simulink model "simModel2020"  (R2023b)
settings: Solver=ode4  StartTime=0  StopTime=360  FixedStep=0.01  RelTol=1e-3
values from neighbouring files (symbols this model uses):
  B747 =     [B747.mat]
undefined symbols (not defined in the file or in its folder): airport, APP, control, Curise, Earth, env, ft, m, navData, navParam, Newton, plotTrack, Raphson, s, TakeOff, WGS84
libraries: aerolibconvert2 x18, simulink x15, sharedtransform x4, aerolibfltsims x3, aerolibatmos2 x2, shared6dof x2, aerolibasang x2, dspsrcs4 x2, aerolibwind2 x2, aerolibanimutils x1, aerolibpropulsion2 x1, aerolibtransform2 x1
(part 2 of 6)

== system simModel2020/PlantModel/Actuator Model/Linear Second-Order Actuator4 ==
  Ac_dem : Inport
  2*zeta * wn : Gain  Gain=2.0 * z_fin* wn_fin  SaturateOnIntegerOverflow=on  OutDataTypeStr=Inherit: Same as input  ParamDataTypeStr=Inherit: Same as input
  "Integrator, Second-Order" : SecondOrderIntegrator  ICX=fin_act_0  UpperLimitX=1  LowerLimitX=0  ICDXDT=fin_act_vel
  Sum2 : Sum  Inputs=|+-  InputSameDT=on  SaturateOnIntegerOverflow=on  OutDataTypeStr=Inherit: Same as first input
  Sum3 : Sum  Inputs=|+-  InputSameDT=on  SaturateOnIntegerOverflow=on  OutDataTypeStr=Inherit: Same as first input
  wn^2 : Gain  Gain=wn_fin* wn_fin  SaturateOnIntegerOverflow=on  OutDataTypeStr=Inherit: Same as input  ParamDataTypeStr=Inherit: Same as input
  Ac_ac : Outport  InitialOutput=0
  wires:
  "Integrator, Second-Order"/1 -> Ac_ac/1, Sum3/2
  wn^2/1 -> Sum2/1
  Sum2/1 -> "Integrator, Second-Order"/1
  2*zeta * wn/1 -> Sum2/2
  Ac_dem/1 -> Sum3/1
  Sum3/1 -> wn^2/1
  "Integrator, Second-Order"/2 -> 2*zeta * wn/1

== system simModel2020/PlantModel/B747 Dynamics动力学参数计算/6DOF Equations of Motion运动学方程 ==
  note: 此处vb为地速ve进行坐标转换得到
  FM_b : Inport
  oil Q : Inport  Port=2
  IsGround : Inport  Port=3
  Deviation On : Inport  Port=4
  6DOF (Euler Angles) : shared6dof/6DOF (Euler Angles)  units=Metric (MKS)  mtype=Fixed  rep=Euler Angles  xme_0=[0 0 0]  Vm_0=[0 0 0]  eul_0=[0 0 0]  pm_0=[0 0 0]  mass_0=1.0  mass_e=0.5  mass_f=2.0  inertia=eye(3)  inertia_e=eye(3)  inertia_f=2*eye(3)  k_quat=1.0  vre_flag=on  abi_flag=off  aMode=0  xme_statename=''  Vm_statename=''  eul_statename=''  quat_statename=''  pm_statename=''  mass_statename=''
  6DOF (Euler Angles)1 : shared6dof/6DOF (Euler Angles)  units=Metric (MKS)  mtype=Simple Variable  rep=Euler Angles  xme_0=B747.ic.Pos_0.*[1; 1; -1]  Vm_0=B747.ic.Vb_0  eul_0=B747.ic.Euler_0  pm_0=B747.ic.PQR_0  mass_0=B747.geometry.mass  mass_e=B747.geometry.massEmpty  mass_f=B747.geometry.massFull  inertia=eye(3)  inertia_e=diag([B747.inertia.Ixx B747.inertia.Iyy B747.inertia.Izz])  inertia_f=diag([B747.inertia.Ixx B747.inertia.Iyy B747.inertia.Izz])  k_quat=1.0  vre_flag=off  abi_flag=off  aMode=aMode  xme_statename=''  Vm_statename=''  eul_statename=''  quat_statename=''  pm_statename=''  mass_statename=''
  Bus Creator : BusCreator  Inputs=8
  Compute psi_dot : Subsystem
  Constant1 : Constant  Value=0
  Demux2 : Demux  Outputs=2
  Multiport Switch : MultiPortSwitch  DataPortOrder=Specify indices  Inputs=[0 1]  DataPortIndices={1,0}  SaturateOnIntegerOverflow=off  InputSameDT=off
  Terminator : Terminator
  Terminator1 : Terminator
  Terminator2 : Terminator
  To Workspace : ToWorkspace  VariableName=Fuel  SampleTime=-1
  "[0, pi] Wrap Around" : Subsystem
  B747 State : Outport
  wires:
  6DOF (Euler Angles)1/8 -> Bus Creator/6  "Ab"
  "[0, pi] Wrap Around"/1(Wrapped) -> Bus Creator/3  "Euler"
  6DOF (Euler Angles)1/5 -> Bus Creator/4  "Vb"
  6DOF (Euler Angles)1/2 -> Bus Creator/2  "Xe"
  6DOF (Euler Angles)1/1 -> Bus Creator/1  "Ve"
  Bus Creator/1 -> B747 State/1
  6DOF (Euler Angles)1/4 -> Terminator1/1
  6DOF (Euler Angles)1/3 -> Compute psi_dot/1(Euler), "[0, pi] Wrap Around"/1(Euler)
  6DOF (Euler Angles)1/6 -> Compute psi_dot/2(G), Bus Creator/5  "pqr"
  FM_b/1 -> Demux2/1
  Demux2/1 -> 6DOF (Euler Angles)1/1
  Compute psi_dot/1(psi_dot) -> Bus Creator/7  "psi_dot"
  Demux2/2 -> 6DOF (Euler Angles)1/2
  Multiport Switch/1 -> 6DOF (Euler Angles)1/3
  Constant1/1 -> Multiport Switch/3
  Deviation On/1 -> Multiport Switch/1
  oil Q/1 -> Multiport Switch/2
  6DOF (Euler Angles)1/9 -> To Workspace/1, Terminator/1
  6DOF (Euler Angles)1/7 -> Terminator2/1
  IsGround/1 -> Bus Creator/8  "IsGround"

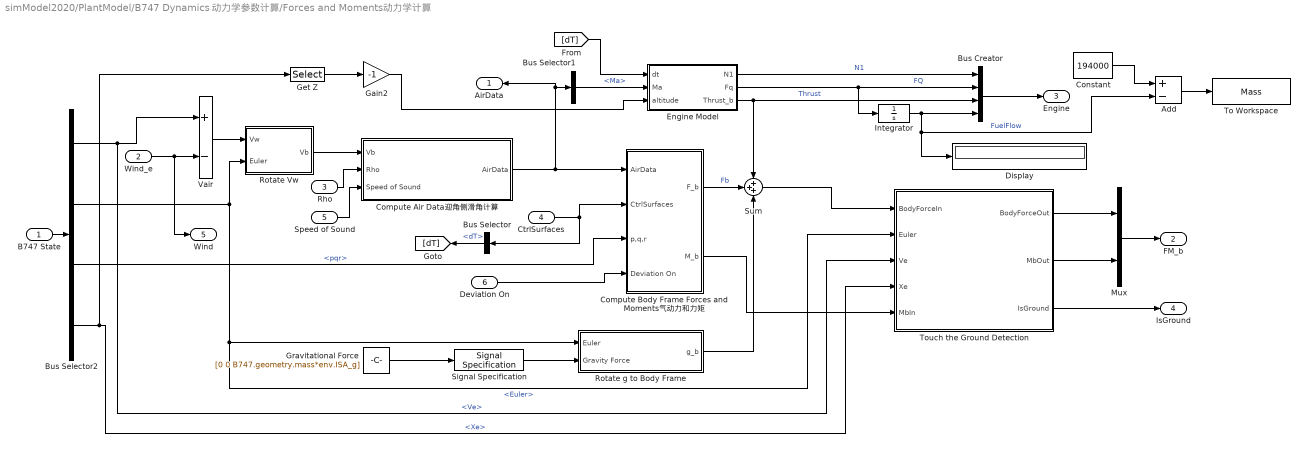
== system simModel2020/PlantModel/B747 Dynamics动力学参数计算/Forces and Moments动力学计算 ==
  B747 State : Inport
  Wind_e : Inport  Port=2
  Rho : Inport  Port=3
  CtrlSurfaces : Inport  Port=4
  Speed of Sound : Inport  Port=5
  Deviation On : Inport  Port=6
  Add : Sum  Inputs=+-
  Bus Creator : BusCreator  Inputs=4
  Bus Selector : BusSelector  OutputSignals=dT
  Bus Selector1 : BusSelector  OutputSignals=Ma
  Bus Selector2 : BusSelector  OutputSignals=Ve,Euler,pqr,Xe
  Compute Air Data迎角侧滑角计算 : Subsystem  TreatAsAtomicUnit=on  VariantControl=use_aerospace_blocks == 1
  Compute Body Frame Forces and Moments气动力和力矩 : Subsystem
  Constant : Constant  Value=194000
  Display : Display
  Engine Model : Subsystem
  Gain2 : Gain  Gain=-1
      settings: AttributesFormatString=Z to Alt
  Get Z : Selector  InputPortWidth=3  IndexOptions=Index vector (dialog)  Indices=[3]  OutputSizes=[(-2)]
  Gravitational Force : Constant  Value=[0 0 B747.geometry.mass*env.ISA_g]  VectorParams1D=off
      settings: AttributesFormatString=%<Value>
  Integrator : Integrator
  Mux : Mux  Inputs=2
  Rotate Vw : Subsystem
  Rotate g to Body Frame : Subsystem
  Signal Specification : SignalSpecification
  Sum : Sum  Inputs=+++  SaturateOnIntegerOverflow=on
  To Workspace : ToWorkspace  VariableName=Mass  SampleTime=-1
  Touch the Ground Detection : Subsystem
  Vair : Sum  Inputs=+-  InputSameDT=on  SaturateOnIntegerOverflow=on  OutDataTypeStr=Inherit: Same as first input
  AirData : Outport
  FM_b : Outport  Port=2
  Engine : Outport  Port=3
  IsGround : Outport  Port=4
  Wind : Outport  Port=5
  wires:
  Bus Selector2/1 -> Touch the Ground Detection/3(Ve), Vair/1  "<Ve>"
  B747 State/1 -> Bus Selector2/1
  Mux/1 -> FM_b/1
  Bus Selector/1 -> [dT]  "<dT>"
  Compute Body Frame Forces and Moments气动力和力矩/1(F_b) -> Sum/2  "Fb"
  Rotate g to Body Frame/1(g_b) -> Sum/3
  Wind_e/1 -> Wind/1, Vair/2
  CtrlSurfaces/1 -> Compute Body Frame Forces and Moments气动力和力矩/2(CtrlSurfaces), Bus Selector/1
  Bus Selector2/3 -> Compute Body Frame Forces and Moments气动力和力矩/3(p,q,r)  "<pqr>"
  Gravitational Force/1 -> Signal Specification/1
  Rotate Vw/1(Vb) -> Compute Air Data迎角侧滑角计算/1(Vb)
  Rho/1 -> Compute Air Data迎角侧滑角计算/2(Rho)
  Bus Selector2/2 -> Rotate Vw/2(Euler), Touch the Ground Detection/2(Euler), Rotate g to Body Frame/1(Euler)  "<Euler>"
  Vair/1 -> Rotate Vw/1(Vw)
  Signal Specification/1 -> Rotate g to Body Frame/2(Gravity Force)
  Touch the Ground Detection/1(BodyForceOut) -> Mux/1
  Sum/1 -> Touch the Ground Detection/1(BodyForceIn)
  Compute Body Frame Forces and Moments气动力和力矩/2(M_b) -> Touch the Ground Detection/5(MbIn)
  Touch the Ground Detection/2(MbOut) -> Mux/2
  Speed of Sound/1 -> Compute Air Data迎角侧滑角计算/3(Speed of Sound)
  Engine Model/1(N1) -> Bus Creator/1  "N1"
  [dT] -> Engine Model/1(dt)
  Engine Model/2(Fq) -> Integrator/1, Bus Creator/2  "FQ"
  Get Z/1 -> Gain2/1
  Bus Selector2/4 -> Get Z/1, Touch the Ground Detection/4(Xe)  "<Xe>"
  Compute Air Data迎角侧滑角计算/1(AirData) -> AirData/1, Bus Selector1/1, Compute Body Frame Forces and Moments气动力和力矩/1(AirData)
  Engine Model/3(Thrust_b) -> Sum/1, Bus Creator/3  "Thrust"
  Bus Selector1/1 -> Engine Model/2(Ma)  "<Ma>"
  Gain2/1 -> Engine Model/3(altitude)
  Deviation On/1 -> Compute Body Frame Forces and Moments气动力和力矩/4(Deviation On)
  Bus Creator/1 -> Engine/1
  Integrator/1 -> Bus Creator/4, Display/1, Add/2  "FuelFlow"
  Touch the Ground Detection/3(IsGround) -> IsGround/1
  Constant/1 -> Add/1
  Add/1 -> To Workspace/1

== system simModel2020/PlantModel/FlightSwitchModel/If Action Subsystem ==
  In1 : Inport
  Action Port : ActionPort  ActionPortLabel=case [ 2 ]:
  Out1 : Outport
  wires:
  In1/1 -> Out1/1

== system simModel2020/PlantModel/FlightSwitchModel/If Action Subsystem1 ==
  CtrlCmds : Inport
  Action Port : ActionPort  ActionPortLabel=case [ 0 ]:
  Out1 : Outport
  wires:
  CtrlCmds/1 -> Out1/1

== system simModel2020/PlantModel/FlightSwitchModel/If Action Subsystem2 ==
  CtrlCmds : Inport
  Action Port : ActionPort  ActionPortLabel=case [ 1 ]:
  Out1 : Outport
  wires:
  CtrlCmds/1 -> Out1/1

== system simModel2020/PlantModel/FlightSwitchModel/Manually piloted aircraft ==
  Gain : Gain  Gain=pi/180
  Gain1 : Gain  Gain=1/100
  Gain2 : Gain  Gain=pi/180
  Gain3 : Gain  Gain=pi/180
  Mux : Mux  Inputs=5
  dA_hand : Constant  Value=16.8
  dE_hand : Constant  Value=-17.3643
  dF_hand : Constant  Value=0
  dR_hand : Constant  Value=-1.3333
  dT_hand : Constant  Value=65.1111
  Out1 : Outport
  wires:
  Mux/1 -> Out1/1
  dR_hand/1 -> Gain3/1
  dA_hand/1 -> Gain2/1
  dE_hand/1 -> Gain/1
  dT_hand/1 -> Gain1/1
  dF_hand/1 -> Mux/5
  Gain/1 -> Mux/1
  Gain1/1 -> Mux/2
  Gain2/1 -> Mux/3
  Gain3/1 -> Mux/4

== system simModel2020/PlantModel/Sensor Model/Assemble GPS and State Data ==
  AirSensorData : Inport
  B747 State : Inport  Port=2
  CtrlSurfaces : Inport  Port=3
  Engine : Inport  Port=4
  Wind : Inport  Port=5
  Bus Creator : BusCreator  Inputs=20
  Bus Selector : BusSelector  OutputSignals=static,q,OAT,airpseed,alpha,beta,Ma,ias
  Bus Selector1 : BusSelector  OutputSignals=dE,dT,dA,dR,dF
  Bus Selector2 : BusSelector  OutputSignals=Euler,pqr,Xe,Ve,Ab,IsGround,Vb
  Bus Selector3 : BusSelector  OutputSignals=Xe
  Bus Selector5 : BusSelector  OutputSignals=N1,FQ
  LLA Position : Subsystem
  Mux : Mux  Inputs=5
  B747 StateBus : Outport
  wires:
  Mux/1 -> Bus Creator/17  "ctrlSurfacePos"
  CtrlSurfaces/1 -> Bus Selector1/1  "ctrlSurfacePos"
  Bus Selector/4 -> Bus Creator/11  "<airpseed>"
  Bus Selector/3 -> Bus Creator/10  "<OAT>"
  Bus Selector/2 -> Bus Creator/9  "<q>"
  Bus Selector/1 -> Bus Creator/8  "<static>"
  Bus Selector2/5 -> Bus Creator/5  "<Ab>"
  Bus Selector2/4 -> Bus Creator/4  "<Ve>"
  Bus Selector2/2 -> Bus Creator/2  "<pqr>"
  Bus Selector2/1 -> Bus Creator/1  "<Euler>"
  Bus Creator/1 -> B747 StateBus/1
  B747 State/1 -> Bus Selector2/1, Bus Selector3/1
  Bus Selector3/1 -> LLA Position/1(XYZ (NEU))  "<Xe>"
  AirSensorData/1 -> Bus Selector/1
  Bus Selector2/3 -> Bus Creator/3  "<Xe>"
  Bus Selector/5 -> Bus Creator/12  "<alpha>"
  Bus Selector/6 -> Bus Creator/13  "<beta>"
  Engine/1 -> Bus Selector5/1  "Engine"
  Bus Selector5/1 -> Bus Creator/18  "<N1>"
  Bus Selector5/2 -> Bus Creator/19  "<FQ>"
  Bus Selector/7 -> Bus Creator/14  "<Ma>"
  Bus Selector/8 -> Bus Creator/15  "<ias>"
  Bus Selector2/6 -> Bus Creator/6  "<IsGround>"
  LLA Position/1(LLA) -> Bus Creator/16  "LLA"
  Bus Selector1/1 -> Mux/1  "<dE>"
  Bus Selector1/2 -> Mux/2  "<dT>"
  Bus Selector1/3 -> Mux/3  "<dA>"
  Bus Selector1/4 -> Mux/4  "<dR>"
  Bus Selector1/5 -> Mux/5  "<dF>"
  Bus Selector2/7 -> Bus Creator/7  "<Vb>"
  Wind/1 -> Bus Creator/20  "Wind"

== system simModel2020/PlantModel/Sensor Model/Noise Model ==
  note: 加速度
  note: 指示空速
  note: 经纬高
  note: 燃油速率
  note: 发动机转速
  note: 操纵面位置
  note: 马赫数
  note: 气流角
  note: 真空速
  note: 外界温度
  note: 动压
  note: 静压
  note: 速度
  note: 位置
  note: 角速率
  note: 欧拉角
  B747 State : Inport
  Bus Creator : BusCreator  Inputs=20
  Bus Selector2 : BusSelector  OutputSignals=Euler,pqr,Xe,Ve,Ab,static,q,OAT,airpseed,alpha,beta,Ma,ctrlSurfacePos,N1,FQ,LLA,ias,IsGround,Vb,Wind
  Gain1 : Gain  Gain=[1 1 -1]
  Gain2 : Gain  Gain=[1 1 -1]
  SensorData : Outport
  wires:
  Bus Creator/1 -> SensorData/1
  Bus Selector2/8 -> Bus Creator/8  "<OAT>"
  Bus Selector2/7 -> Bus Creator/7  "<q>"
  Bus Selector2/6 -> Bus Creator/6  "<static>"
  Bus Selector2/4 -> Gain1/1  "<Ve>"
  Bus Selector2/1 -> Bus Creator/1  "<Euler>"
  B747 State/1 -> Bus Selector2/1
  Bus Selector2/10 -> Bus Creator/10  "<alpha>"
  Bus Selector2/3 -> Gain2/1  "<Xe>"
  Bus Selector2/5 -> Bus Creator/5  "<Ab>"
  Bus Selector2/9 -> Bus Creator/9  "<airpseed>"
  Bus Selector2/2 -> Bus Creator/2  "<pqr>"
  Gain2/1 -> Bus Creator/3  "Xe"
  Gain1/1 -> Bus Creator/4  "Ve"
  Bus Selector2/11 -> Bus Creator/11  "<beta>"
  Bus Selector2/12 -> Bus Creator/12  "<Ma>"
  Bus Selector2/13 -> Bus Creator/13  "<ctrlSurfacePos>"
  Bus Selector2/14 -> Bus Creator/14  "<N1>"
  Bus Selector2/15 -> Bus Creator/15  "<FQ>"
  Bus Selector2/16 -> Bus Creator/16  "<LLA>"
  Bus Selector2/17 -> Bus Creator/17  "<ias>"
  Bus Selector2/18 -> Bus Creator/18  "<IsGround>"
  Bus Selector2/19 -> Bus Creator/19  "<Vb>"
  Bus Selector2/20 -> Bus Creator/20  "<Wind>"

== system simModel2020/PlantModel/Wind Model/ Compute Norm ==
  V : Inport
  Dot Product : DotProduct  OutDataTypeStr=Inherit: Inherit via internal rule
  Math Function1 : Sqrt  AlgorithmType=Newton-Raphson
      settings: AttributesFormatString=%<AlgorithmType>
  Zero Bound : Saturate  UpperLimit=inf  LowerLimit=0.001
      settings: AttributesFormatString="[%<LowerLimit>  %<UpperLimit>]"
  |V| : Outport
  wires:
  Math Function1/1 -> |V|/1
  V/1 -> Dot Product/2, Dot Product/1
  Dot Product/1 -> Zero Bound/1
  Zero Bound/1 -> Math Function1/1

== system simModel2020/PlantModel/Wind Model/Average wind ==
  DCM : Inport
  " " : Gain  Gain=-1  SaturateOnIntegerOverflow=on  OutDataTypeStr=Inherit: Same as input  ParamDataTypeStr=Inherit: Same as input
  Angle Conversion : aerolibconvert2/Angle Conversion  IU=deg  OU=rad
  Mux : Mux  Inputs=3
  Product1 : Product  InputSameDT=on  SaturateOnIntegerOverflow=on  OutDataTypeStr=Inherit: Same as first input
  SinCos : Trigonometry  Operator=sincos
  Transform from Inertial to Body axes : Product  Inputs=**  Multiplication=Matrix(*)  InputSameDT=on  SaturateOnIntegerOverflow=on  OutDataTypeStr=Inherit: Same as first input
  Wdeg1 : Constant  Value=0  OutDataTypeStr=Inherit: Inherit via back propagation
  Wind Direction : Constant  Value=Wdeg  OutDataTypeStr=Inherit: Inherit via back propagation
  Wind Speed : Constant  Value=Vwind  OutDataTypeStr=Inherit: Inherit via back propagation
  Wind Velocity : Outport
  wires:
  " "/1 -> Product1/2
  DCM/1 -> Transform from Inertial to Body axes/1
  Mux/1 -> " "/1
  Transform from Inertial to Body axes/1 -> Wind Velocity/1
  SinCos/1 -> Mux/2  "Wy"
  Angle Conversion/1 -> SinCos/1
  Wind Speed/1 -> Product1/1
  SinCos/2 -> Mux/1  "Wx"
  Product1/1 -> Transform from Inertial to Body axes/2
  Wdeg1/1 -> Mux/3  "Wz"
  Wind Direction/1 -> Angle Conversion/1

== system simModel2020/PlantModel/Wind Model/RL2B ==
  Euler : Inport
  Rotation Angles to Direction Cosine Matrix1 : sharedtransform/Rotation Angles to Direction Cosine Matrix  rotationOrder=ZYX  aMode=aMode
  Selector : Selector  InputPortWidth=3  IndexOptions=Index vector (dialog)  Indices=[3 2 1]  OutputSizes=1
  RL2B : Outport
  wires:
  Rotation Angles to Direction Cosine Matrix1/1 -> RL2B/1
  Euler/1 -> Selector/1
  Selector/1 -> Rotation Angles to Direction Cosine Matrix1/1

== system simModel2020/PlantModel/Wind Model/Random wind ==
  DCM : Inport
  " 1" : Gain  Gain=-1  SaturateOnIntegerOverflow=on  OutDataTypeStr=Inherit: Same as input  ParamDataTypeStr=Inherit: Same as input
  Constant : Constant  Value=90
  Math Function : Math  Operator=transpose  SignedPower=on
  Mux : Mux  Inputs=3
  Product : Product
  Product1 : Product  InputSameDT=on  SaturateOnIntegerOverflow=on  OutDataTypeStr=Inherit: Same as first input
  Product3 : Product
  SinCos : Trigonometry  Operator=sincos
  SinCos1 : Trigonometry  Operator=sincos
  Transform from Inertial to Body axes : Product  Inputs=**  Multiplication=Matrix(*)  InputSameDT=on  SaturateOnIntegerOverflow=on  OutDataTypeStr=Inherit: Same as first input
  Wind speed : dspsrcs4/Random Source  SrcType=Gaussian  NormMethod=Ziggurat  CltLength=12  MinVal=0  MaxVal=1  MeanVal=[mu(1) mu(2) mu(3)]  VarVal=[(sigma(1))^2 (sigma(2))^2 (sigma(3))^2]  RepMode=Not repeatable  rawSeed=1  IsInherit=off  SampMode=Continuous  SampTime=1  SampFrame=1  DataType=Double  OutComplex=Real  OutputFrames=on
  wind direction J_2(rad) : dspsrcs4/Random Source  SrcType=Uniform  NormMethod=Ziggurat  CltLength=12  MinVal=0  MaxVal=2*pi  MeanVal=0  VarVal=1  RepMode=Not repeatable  rawSeed=1  IsInherit=off  SampMode=Continuous  SampTime=1  SampFrame=1  DataType=Double  OutComplex=Real  OutputFrames=on
  u_w,v_w,w_w (m/s) : Outport
  wires:
  Constant/1 -> SinCos1/1
  " 1"/1 -> Product1/2
  SinCos1/2 -> Mux/3
  wind direction J_2(rad)/1 -> SinCos/1
  Product/1 -> Mux/2
  SinCos/2 -> Product3/1
  Mux/1 -> " 1"/1
  SinCos/1 -> Product/1
  SinCos1/1 -> Product3/2, Product/2
  Product3/1 -> Mux/1
  Wind speed/1 -> Product1/1
  Transform from Inertial to Body axes/1 -> Math Function/1
  DCM/1 -> Transform from Inertial to Body axes/2
  Product1/1 -> Transform from Inertial to Body axes/1
  Math Function/1 -> u_w,v_w,w_w (m/s)/1

== system simModel2020/PlantModel/Wind Model/Vonkarman Turbulence ==
  Altitude(m) : Inport
  Airspeed(m/s) : Inport  Port=2
  DCM : Inport  Port=3  PortDimensions=[3 3]
  (u,v,w) : Selector  InputPortWidth=3  IndexOptions=Index vector (dialog)  Indices=[1 2 3]  OutputSizes=1
  Angle Conversion1 : aerolibconvert2/Angle Conversion  IU=deg  OU=rad
  Band-Limited White Noise : simulink/Sources/Band-Limited White Noise  Cov=[1 1 1]*pi  Ts=ts  seed=Seed
  Bus Creator : BusCreator  Inputs=3
  Filters on velocities : Subsystem
  Mux : Mux  Inputs=3
  Select velocities : aerolibwind2/Dryden Wind Turbulence Model  (Continuous (+q -r))/Select velocities  SystemSampleTime=-1  VariantActivationTime=update diagram  AllowFlexibleInterface=on  Latency=0  AutoFrameSizeCalculation=off
  Turbulence intensities : aerolibwind2/Dryden Wind Turbulence Model  (Continuous (+q -r))/RMS turbulence  intensities  SystemSampleTime=-1  VariantActivationTime=update diagram  AllowFlexibleInterface=on  Latency=0  AutoFrameSizeCalculation=off
  Turbulence scale lengths : Subsystem
  Velocity Conversion : aerolibconvert2/Velocity Conversion  IU=m/s  OU=ft/s
  Velocity Conversion1 : aerolibconvert2/Velocity Conversion  IU=m/s  OU=ft/s
  Velocity Conversion2 : aerolibconvert2/Velocity Conversion  IU=ft/s  OU=m/s
  Wind direction : Constant  Value=Wdeg  OutDataTypeStr=Inherit: Inherit via back propagation
  Windspeed at 20ft (6m) : Constant  Value=W20  OutDataTypeStr=Inherit: Inherit via back propagation
  u_w,v_w,w_w (m/s) : Outport
  wires:
  Velocity Conversion2/1 -> u_w,v_w,w_w (m/s)/1
  Mux/1 -> Velocity Conversion2/1
  Windspeed at 20ft (6m)/1 -> Velocity Conversion/1
  (u,v,w)/1 -> Filters on velocities/1(Noise)
  Bus Creator/1 -> Select velocities/1
  Velocity Conversion1/1 -> Filters on velocities/8(V)
  Filters on velocities/2(vgw) -> Select velocities/3  "vgw"
  Angle Conversion1/1 -> Bus Creator/2  "Wdeg"
  Turbulence scale lengths/1(L_ug) -> Filters on velocities/2(L_ug)
  Band-Limited White Noise/1 -> (u,v,w)/1
  Turbulence intensities/3 -> Filters on velocities/7(sigma_wg)
  Turbulence intensities/1 -> Filters on velocities/5(sigma_ug)
  Altitude(m)/1 -> Turbulence intensities/1, Bus Creator/3, Turbulence scale lengths/1(Altitude)  "altitude"
  Turbulence scale lengths/2(L_vg) -> Filters on velocities/3(L_vg)
  Select velocities/2 -> Mux/2
  Filters on velocities/1(ugw) -> Select velocities/2  "ugw"
  Select velocities/3 -> Mux/3
  Turbulence intensities/2 -> Filters on velocities/6(sigma_vg)
  Filters on velocities/3(wgw) -> Select velocities/4  "wgw"
  Airspeed(m/s)/1 -> Velocity Conversion1/1
  Wind direction/1 -> Angle Conversion1/1
  Select velocities/1 -> Mux/1
  Turbulence scale lengths/3(L_wg) -> Filters on velocities/4(L_wg)
  DCM/1 -> Bus Creator/1  "DCM"
  Velocity Conversion/1 -> Turbulence intensities/2

== system simModel2020/PlantModel/Wind Model/Wind Shear ==
  Altitude(m) : Inport
  DCM : Inport  Port=2  PortDimensions=[3 3]
  3ft-->inf : Saturate  UpperLimit=inf  LowerLimit=3
  Angle Conversion : aerolibconvert2/Angle Conversion  IU=deg  OU=rad
  Length Conversion : aerolibconvert2/Length Conversion  IU=m  OU=ft
  Mux : Mux  Inputs=3
  Product : Product  Inputs=*/  InputSameDT=on  SaturateOnIntegerOverflow=on  OutDataTypeStr=Inherit: Same as first input
  Product1 : Product  InputSameDT=on  SaturateOnIntegerOverflow=on  OutDataTypeStr=Inherit: Same as first input
  Reshape : Reshape  OutputDimensionality=Column vector (2-D)
  Reshape1 : Reshape
  SinCos : Trigonometry  Operator=sincos
  Transform from Inertial to Body axes : Product  Inputs=**  Multiplication=Matrix(*)  InputSameDT=on  SaturateOnIntegerOverflow=on  OutDataTypeStr=Inherit: Same as first input
  Wdeg1 : Constant  Value=0  OutDataTypeStr=Inherit: Inherit via back propagation
  Wind Direction : Constant  Value=Wdeg  OutDataTypeStr=Inherit: Inherit via back propagation
  Wind speed at reference height : Gain  Gain=-W_20  SaturateOnIntegerOverflow=on  OutDataTypeStr=Inherit: Same as input  ParamDataTypeStr=Inherit: Same as input
  h/z0 : Gain  Gain=1/z0  SaturateOnIntegerOverflow=on  OutDataTypeStr=Inherit: Same as input  ParamDataTypeStr=Inherit: Same as input
  ln(h/z0) : Math  Operator=log  SignedPower=on
  ln(ref_height/z0) : Math  Operator=log  SignedPower=on
  ref_height/z0 : Constant  Value=20/z0  OutDataTypeStr=Inherit: Inherit via back propagation
  u_w,v_w,w_w (m/s) : Outport
  wires:
  ln(ref_height/z0)/1 -> Product/2
  Product1/1 -> Reshape/1
  Reshape1/1 -> u_w,v_w,w_w (m/s)/1
  Wind Direction/1 -> Angle Conversion/1
  Reshape/1 -> Transform from Inertial to Body axes/2
  Altitude(m)/1 -> Length Conversion/1
  h/z0/1 -> ln(h/z0)/1
  Angle Conversion/1 -> SinCos/1
  Length Conversion/1 -> 3ft-->inf/1
  SinCos/2 -> Mux/1  "Wx"
  ln(h/z0)/1 -> Product/1
  DCM/1 -> Transform from Inertial to Body axes/1
  3ft-->inf/1 -> h/z0/1
  Product/1 -> Product1/1
  ref_height/z0/1 -> ln(ref_height/z0)/1
  SinCos/1 -> Mux/2  "Wy"
  Wind speed at reference height/1 -> Product1/2
  Wdeg1/1 -> Mux/3  "Wz"
  Transform from Inertial to Body axes/1 -> Reshape1/1
  Mux/1 -> Wind speed at reference height/1

== system simModel2020/AutoPilot/InnerLoopAutopilot/Latitudinal Channel维度通道/Eliminate sideslip ==
  <beta> : Inport
  <Ab> : Inport  Port=2
  Data Type Conversion : DataTypeConversion  SaturateOnIntegerOverflow=off  RndMeth=Floor
  Gain3 : Gain  Gain=-5
  Gain4 : Gain  Gain=0.05
  Neg Feedback : Gain  Gain=-1  OutDataTypeStr=float('double')
      settings: AttributesFormatString=%<Gain>
  Selector3 : Selector  InputPortWidth=3  IndexOptions=Index vector (dialog)  Indices=[2]  OutputSizes=1
  Sum1 : Sum  Inputs=++|
  "[-20 20]" : Saturate  UpperLimit=20  LowerLimit=-20
      settings: AttributesFormatString="[%<LowerLimit>  %<UpperLimit>]"
  dR : Outport
  wires:
  Neg Feedback/1 -> Gain4/1
  <beta>/1 -> Gain3/1
  "[-20 20]"/1 -> Neg Feedback/1
  Gain4/1 -> Sum1/2
  Selector3/1 -> "[-20 20]"/1
  Sum1/1 -> Data Type Conversion/1
  <Ab>/1 -> Selector3/1  "Ab"
  Data Type Conversion/1 -> dR/1
  Gain3/1 -> Sum1/1

== system simModel2020/AutoPilot/InnerLoopAutopilot/Latitudinal Channel维度通道/Lateral Correction ==
  y : Inport
  psi_c : Inport  Port=2
  psi : Inport  Port=3
  Roll(k-1) : Inport  Port=4
  Action Port : ActionPort  ActionPortLabel=case [ 1 ]:
  Add : Sum  Inputs=+-
  Clock : Clock
  Filter1 : Subsystem
  Gain : Gain  Gain=-0.0002
  Gain1 : Gain  Gain=2
  MATLAB Function : MATLAB Function  TreatAsAtomicUnit=on
  Mux : Mux  Inputs=2
  Scope4 : Scope
  Selector : Selector  InputPortWidth=3  IndexOptions=Index vector (dialog)  Indices=[ 3]  OutputSizes=1
  Sum : Sum  Inputs=|++
  y_c : Constant  Value=0
  Roll_Cmd : Outport
  wires:
  Sum/1 -> Filter1/1(x)
  Roll(k-1)/1 -> Filter1/2(SW_x(k-1))
  Clock/1 -> Filter1/3(time)
  Add/1 -> Gain/1
  y/1 -> Mux/2, Add/2
  psi/1 -> Selector/1
  Selector/1 -> MATLAB Function/2(psi)
  MATLAB Function/1(Psi_Error) -> Gain1/1
  Gain1/1 -> Sum/2
  Gain/1 -> Sum/1
  psi_c/1 -> MATLAB Function/1(psi_c)
  y_c/1 -> Mux/1, Add/1  "cmd_h"
  Mux/1 -> Scope4/1
  Filter1/1(y) -> Roll_Cmd/1

== system simModel2020/AutoPilot/InnerLoopAutopilot/Latitudinal Channel维度通道/Roll Control ==
  phi_c : Inport
  phi : Inport  Port=2
  pqr : Inport  Port=3
  Roll(k-1) : Inport  Port=4
  Add : Sum  Inputs=+-
  Clock : Clock
  Filter1 : Subsystem
  Gain : Gain  Gain=-10
  Gain1 : Gain  Gain=4
  Selector : Selector  InputPortWidth=3  IndexOptions=Index vector (dialog)  Indices=[ 1]  OutputSizes=1
  Selector1 : Selector  InputPortWidth=3  IndexOptions=Index vector (dialog)  Indices=[ 1]  OutputSizes=1
  Sum : Sum  Inputs=|++
  dA : Outport
  wires:
  Roll(k-1)/1 -> Filter1/2(SW_x(k-1))
  Clock/1 -> Filter1/3(time)
  Selector1/1 -> Gain1/1
  Gain/1 -> Sum/1
  phi/1 -> Selector/1
  Gain1/1 -> Sum/2
  Add/1 -> Gain/1
  pqr/1 -> Selector1/1
  phi_c/1 -> Add/1  "cmd_h"
  Selector/1 -> Add/2  "phi"
  Sum/1 -> Filter1/1(x)
  Filter1/1(y) -> dA/1

== system simModel2020/AutoPilot/InnerLoopAutopilot/Latitudinal Channel维度通道/Roll Hold ==
  phi_cmd : Inport
  Action Port : ActionPort  InitializeStates=reset  ActionPortLabel=case [ 2 ]:
  Roll_Cmd : Outport
  wires:
  phi_cmd/1 -> Roll_Cmd/1

== system simModel2020/AutoPilot/InnerLoopAutopilot/Latitudinal Channel维度通道/Sample(1//z) ==
  <Mode> : Inport
  x : Inport  Port=2
  Detect Change : Subsystem  mask(Detect Change){vinit=0, InputProcessing=Elements as channels (sample based), OutDataTypeStr=boolean}
      mask prompts: vinit "Simulink:masks:InitialCondition_MP"; InputProcessing "Simulink:masks:InputProcessing_MP"; OutDataTypeStr "Simulink:masks:OutputDataType_MP"
      mask help: Simulink:masks:DetectChange_MD
      mask init:
      | initDetectBlocks();
      mask TypeOptions InputProcessing: Simulink:masks:ColumnsAsChannelsFrameBased | Simulink:masks:ElementsAsChannelsSampleBased
      mask TypeOptions OutDataTypeStr: Simulink:masks:uint8 | Simulink:masks:boolean
      mask Display: fprintf('U ~= U/z')
  Sample and Hold : Subsystem  TreatAsAtomicUnit=on  mask(Sample and Hold){trig=Either edge, initCond=0, latchinput=off}
      mask prompts: trig "Trigger type:"; initCond "Initial condition:"; latchinput "Latch (buffer) input"
      mask help: Sample and hold the input signal. If Latch (buffer) input is selected, then this block produces the value of the input from the previous time step.
      mask init:
      | switch trig
      | case 1, s='rising';
      | case 2, s='falling';
      | case 3, s='either';
      | end
      | set_param([gcb '/Trigger'],'triggertype',s);
      | if (latchinput == 1)
      | 	set_param([gcb '/In'],'latchinput','on');
      | else
      | 	set_param([gcb '/In'],'latchinput','off');
      | end
      mask Help: eval('blocksethelp');
      mask TypeOptions trig: Rising edge | Falling edge | Either edge
      mask Display: disp('S/H')
  Unit Delay : UnitDelay  SampleTime=-1  HasFrameUpgradeWarning=on
  y : Outport
  wires:
  <Mode>/1 -> Detect Change/1(U)
  Detect Change/1(Y) -> Sample and Hold/Trigger
  x/1 -> Unit Delay/1
  Unit Delay/1 -> Sample and Hold/1(In)
  Sample and Hold/1(" ") -> y/1

== system simModel2020/AutoPilot/InnerLoopAutopilot/Latitudinal Channel维度通道/Yaw Select ==
  psi_c : Inport
  psi : Inport  Port=2
  Roll(k-1) : Inport  Port=3
  Action Port : ActionPort  ActionPortLabel=case [ 3 ]:
  Clock : Clock
  Filter1 : Subsystem
  Gain1 : Gain  Gain=0.5
  MATLAB Function : MATLAB Function  TreatAsAtomicUnit=on
  Selector : Selector  InputPortWidth=3  IndexOptions=Index vector (dialog)  Indices=[ 3]  OutputSizes=1
  Roll_Cmd : Outport
  wires:
  psi/1 -> Selector/1
  Clock/1 -> Filter1/3(time)
  Roll(k-1)/1 -> Filter1/2(SW_x(k-1))
  MATLAB Function/1(Psi_Error) -> Gain1/1
  Gain1/1 -> Filter1/1(x)
  Filter1/1(y) -> Roll_Cmd/1
  Selector/1 -> MATLAB Function/2(psi)
  psi_c/1 -> MATLAB Function/1(psi_c)

== system simModel2020/AutoPilot/InnerLoopAutopilot/Longitudinal Channel经度通道/AutoThrottle ==
  note: AT_Mode =0: 回收方式
      | AT_Mode =1: 油门保持
      | AT_Mode =2: 速度油门控制
      | AT_Mode =3: 推力控制
      | AT_Mode =4: 预位方式
      | AT_Mode =5: 怠速状态
  APCommands : Inport
  N1 : Inport  Port=2
  <ias> : Inport  Port=3
  AT Mode = 0,Recycle : Subsystem  TreatAsAtomicUnit=on
  AT Mode = 2,MCP Speed : Subsystem  TreatAsAtomicUnit=on
  AT Mode = 3,Throttle Control : Subsystem  TreatAsAtomicUnit=on
  AT Mode = 5,Idle : Subsystem  TreatAsAtomicUnit=on
  Bus Selector : BusSelector  OutputSignals=AT_Mode,IAS_Cmd,N1_Cmd
  Clock : Clock
  Multiport Switch : MultiPortSwitch  DataPortOrder=Zero-based contiguous  Inputs=6  zeroidx=on  SaturateOnIntegerOverflow=off  InputSameDT=off
  Sample(1/z) : Subsystem
  Switch Case : SwitchCase  CaseConditions={0,2,3,5}  ShowDefaultCase=off
  Throttle Limit : Saturate  UpperLimit=control.dtLimit  LowerLimit=B747.engine.Idle
      settings: AttributesFormatString="[%<LowerLimit>  %<UpperLimit>]"
  dT : Outport
  wires:
  <ias>/1 -> AT Mode = 2,MCP Speed/3(<ias>)
  APCommands/1 -> Bus Selector/1
  Bus Selector/1 -> Multiport Switch/1, Sample(1/z)/1(<AT_Mode>), Switch Case/1  "<AT_Mode>"
  Bus Selector/3 -> AT Mode = 3,Throttle Control/1(N1_Cmd)  "<N1_Cmd>"
  AT Mode = 2,MCP Speed/1(dT) -> Multiport Switch/4
  AT Mode = 3,Throttle Control/1(dT) -> Multiport Switch/5
  Switch Case/2 -> AT Mode = 2,MCP Speed/Action
  Switch Case/3 -> AT Mode = 3,Throttle Control/Action
  Bus Selector/2 -> AT Mode = 2,MCP Speed/1(<U_c>)  "<IAS_Cmd>"
  AT Mode = 0,Recycle/1(dT) -> Multiport Switch/2
  Multiport Switch/1 -> Throttle Limit/1
  N1/1 -> AT Mode = 3,Throttle Control/2(N1), AT Mode = 2,MCP Speed/2(N1)
  Sample(1/z)/1(y) -> AT Mode = 2,MCP Speed/4(dT(k-1)), AT Mode = 5,Idle/1(dT(k-1)), AT Mode = 3,Throttle Control/3(dT(k-1)), Multiport Switch/6, Multiport Switch/3, AT Mode = 0,Recycle/1(dT(k-1))
  Switch Case/1 -> AT Mode = 0,Recycle/Action
  Clock/1 -> AT Mode = 5,Idle/2(time), AT Mode = 0,Recycle/2(time), AT Mode = 2,MCP Speed/5(time), AT Mode = 3,Throttle Control/4(time)
  AT Mode = 5,Idle/1(dT) -> Multiport Switch/7
  Switch Case/4 -> AT Mode = 5,Idle/Action
  Throttle Limit/1 -> Sample(1/z)/2(x), dT/1

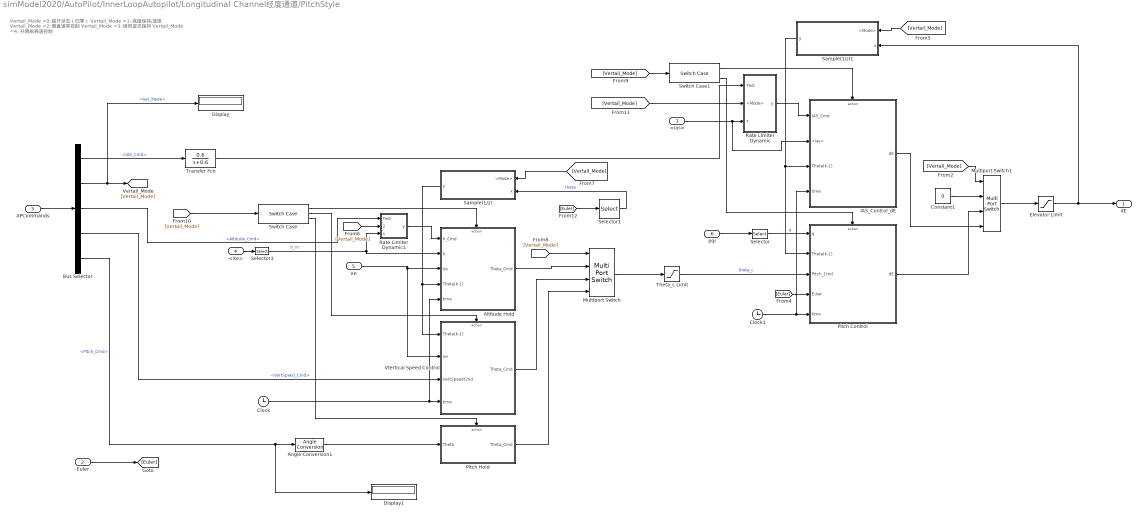
== system simModel2020/AutoPilot/InnerLoopAutopilot/Longitudinal Channel经度通道/PitchStyle ==
  note: Vertail_Mode =0: 脱开状态（归零）
      | Vertail_Mode =1: 高度保持/选择
      | Vertail_Mode =2: 垂直速率控制
      | Vertail_Mode =3: 俯仰姿态保持
      | Vertail_Mode =4: 升降舵表速控制
  <ias> : Inport
  Euler : Inport  Port=2
  APCommands : Inport  Port=3
  <Xe> : Inport  Port=4
  Ve : Inport  Port=5
  pqr : Inport  Port=6
  Altitude Hold : Subsystem  TreatAsAtomicUnit=on
  Angle Conversion1 : aerolibconvert2/Angle Conversion  IU=deg  OU=rad
  Bus Selector : BusSelector  OutputSignals=IAS_Cmd,Ver_Mode,Altitude_Cmd,VertSpeed_Cmd,Pitch_Cmd
  Clock : Clock
  Clock1 : Clock
  Constant1 : Constant  Value=0
  Display : Display
  Display1 : Display
  Elevator Limit : Saturate  UpperLimit=control.deLimit  LowerLimit=-control.deLimit
      settings: AttributesFormatString="[%<LowerLimit>  %<UpperLimit>]"
  IAS_Control_dE : Subsystem  TreatAsAtomicUnit=on
  Multiport Switch : MultiPortSwitch  DiagnosticForDefault=None  SaturateOnIntegerOverflow=off  InputSameDT=off
  Multiport Switch1 : MultiPortSwitch  DataPortOrder=Specify indices  Inputs=2  DataPortIndices={0,[1,2,3],4}  DiagnosticForDefault=None  SaturateOnIntegerOverflow=off  InputSameDT=off
  Pitch Control : Subsystem  TreatAsAtomicUnit=on
  Pitch Hold : Subsystem  TreatAsAtomicUnit=on
  Rate Limiter Dynamic : Subsystem
  Rate Limiter Dynamic1 : Subsystem
  Sample(1/z) : Subsystem
  Sample(1/z)1 : Subsystem
  Selector : Selector  InputPortWidth=3  IndexOptions=Index vector (dialog)  Indices=[2]  OutputSizes=1
  Selector1 : Selector  InputPortWidth=3  IndexOptions=Index vector (dialog)  Indices=[2]  OutputSizes=1
  Selector3 : Selector  InputPortWidth=3  IndexOptions=Index vector (dialog)  Indices=[3]  OutputSizes=1
  Switch Case : SwitchCase  CaseConditions={1,2,3}  ShowDefaultCase=off
  Switch Case1 : SwitchCase  CaseConditions={0}
  Theta_c Limit : Saturate  UpperLimit=control.theta_Limit  LowerLimit=-control.theta_Limit
      settings: AttributesFormatString="[%<LowerLimit>  %<UpperLimit>]"
  Transfer Fcn : TransferFcn  Numerator=[0.6]  Denominator=[1 0.6]
  Vtertical Speed Control : Subsystem  TreatAsAtomicUnit=on
  dE : Outport
  wires:
  Ve/1 -> Altitude Hold/3(Ve), Vtertical Speed Control/2(Ve)
  [Euler] -> Pitch Control/4(Euler)
  Euler/1 -> [Euler]
  APCommands/1 -> Bus Selector/1
  Bus Selector/4 -> Vtertical Speed Control/3(VertSpeedCmd)  "<VertSpeed_Cmd>"
  pqr/1 -> Selector/1
  Selector/1 -> Pitch Control/1(q)  "q"
  Vtertical Speed Control/1(Theta_Cmd) -> Multiport Switch/3
  Theta_c Limit/1 -> Pitch Control/3(Pitch_Cmd)  "theta_c"
  <ias>/1 -> IAS_Control_dE/2(<ias>), Rate Limiter Dynamic/3(x)
  Bus Selector/1 -> Transfer Fcn/1  "<IAS_Cmd>"
  Multiport Switch/1 -> Theta_c Limit/1
  Altitude Hold/1(Theta_Cmd) -> Multiport Switch/2
  Multiport Switch1/1 -> Elevator Limit/1
  Elevator Limit/1 -> Sample(1/z)1/2(x), dE/1
  Switch Case/1 -> Altitude Hold/Action
  Switch Case1/1 -> IAS_Control_dE/Action
  Sample(1/z)1/1(y) -> Pitch Control/2(Theta(k-1)), IAS_Control_dE/3(Theta(k-1))
  Switch Case1/2 -> Pitch Control/Action
  Rate Limiter Dynamic/1(y) -> IAS_Control_dE/1(IAS_Cmd)
  <Xe>/1 -> Selector3/1
  Selector3/1 -> Rate Limiter Dynamic1/3(x), Altitude Hold/2(h)  "h_m"
  Bus Selector/2 -> Display/1, [Vertail_Mode]  "<Ver_Mode>"
  [Vertail_Mode] -> Multiport Switch1/1
  [Vertail_Mode] -> Sample(1/z)1/1(<Mode>)
  [Vertail_Mode] -> Sample(1/z)/1(<Mode>)
  [Vertail_Mode] -> Multiport Switch/1
  [Vertail_Mode] -> Switch Case1/1
  [Vertail_Mode] -> Switch Case/1
  Sample(1/z)/1(y) -> Vtertical Speed Control/1(Theta(k-1)), Altitude Hold/4(Theta(k-1))
  Pitch Hold/1(Theta_Cmd) -> Multiport Switch/4
  Switch Case/3 -> Pitch Hold/Action
  [Vertail_Mode] -> Rate Limiter Dynamic/2(<Mode>)
  Transfer Fcn/1 -> Rate Limiter Dynamic/1(Test)
  Switch Case/2 -> Vtertical Speed Control/Action
  [Vertail_Mode] -> Rate Limiter Dynamic1/2(<Mode>)
  Bus Selector/3 -> Rate Limiter Dynamic1/1(Test)  "<Altitude_Cmd>"
  Constant1/1 -> Multiport Switch1/2
  IAS_Control_dE/1(dE) -> Multiport Switch1/4
  Pitch Control/1(dE) -> Multiport Switch1/3
  [Euler] -> Selector1/1
  Selector1/1 -> Sample(1/z)/2(x)  "theta"
  Clock/1 -> Altitude Hold/5(time), Vtertical Speed Control/4(time)
  Clock1/1 -> IAS_Control_dE/4(time), Pitch Control/5(time)
  Bus Selector/5 -> Display1/1, Angle Conversion1/1  "<Pitch_Cmd>"
  Angle Conversion1/1 -> Pitch Hold/1(Theta)
  Rate Limiter Dynamic1/1(y) -> Altitude Hold/1(h_Cmd)

== system simModel2020/PlantModel/B747 Dynamics动力学参数计算/6DOF Equations of Motion运动学方程/Compute psi_dot ==
  Euler : Inport
  G : Inport  Port=2
  Mux1 : Mux  Inputs=2
  psidot : Fcn  Expr=(u[5]*sin(u[1])+u[6]*cos(u[1]))/cos(u[2])
  psi_dot : Outport
  wires:
  G/1 -> Mux1/2
  psidot/1 -> psi_dot/1  "psi_dot"
  Mux1/1 -> psidot/1
  Euler/1 -> Mux1/1

== system simModel2020/PlantModel/B747 Dynamics动力学参数计算/6DOF Equations of Motion运动学方程/[0, pi] Wrap Around ==
  Euler : Inport
  Compare To Zero : Subsystem  mask(Compare To Zero){relop=>=, OutDataTypeStr=uint8, ZeroCross=off}
      mask prompts: relop "Simulink:masks:Operator_MP"; OutDataTypeStr "Simulink:masks:OutputDataType_MP"; ZeroCross "Simulink:masks:EnableZerocrossingDetection_MP"
      mask help: Simulink:masks:CompareToZero_MD
      mask init:
      | blkName = gcb;
      | 
      | if strcmp(get_param(gcbh,'OutDataTypeStr'),'boolean')
      | 	setValue = 'boolean';
      | else
      |     setValue = 'fixdt(0, 8)';
      | end
      | 
      | set_param([blkName,'/Compare'],'relop',relop, ...
      | 	'OutDataTypeStr', setValue, 'ZeroCross', ZeroCross);
      mask TypeOptions relop: == | ~= | < | <= | >= | >
      mask TypeOptions OutDataTypeStr: Simulink:masks:uint8 | Simulink:masks:boolean
      mask Callback ZeroCross: sl('zeroCrossEnable', gcbh);
      mask Display: disp([relop,' 0'])
  Logical Operator : Logic  Operator=NOT  AllPortsSameDT=off  OutDataTypeStr=boolean
  Merge : Merge  InitialOutput=0
  Mux2 : Mux  Inputs=2
  Negative Yaw : Subsystem
  Positive Yaw : Subsystem
  Selector1 : Selector  InputPortWidth=3  IndexOptions=Index vector (dialog)  Indices=[1 2]  OutputSizes=1
  Selector2 : Selector  InputPortWidth=3  IndexOptions=Index vector (dialog)  Indices=[3]  OutputSizes=1
  Wrapped : Outport
  wires:
  Negative Yaw/1(yaw_wr) -> Merge/2
  Positive Yaw/1(yaw_wr) -> Merge/1
  Merge/1 -> Mux2/2
  Logical Operator/1 -> Negative Yaw/Enable
  Compare To Zero/1(y) -> Logical Operator/1, Positive Yaw/Enable
  Selector2/1 -> Negative Yaw/1(yaw), Positive Yaw/1(yaw), Compare To Zero/1(u)
  Mux2/1 -> Wrapped/1
  Selector1/1 -> Mux2/1
  Euler/1 -> Selector1/1, Selector2/1

== system simModel2020/PlantModel/B747 Dynamics动力学参数计算/Forces and Moments动力学计算/Compute Air Data迎角侧滑角计算 ==
  Vb : Inport  PortDimensions=3
  Rho : Inport  Port=2
  Speed of Sound : Inport  Port=3
  " " : aerolibasang/Incidence, Sideslip, & Airspeed
  Bus Creator : BusCreator  Inputs=5
  Dynamic Pressure动压 : Subsystem  mask(Dynamic Pressure){}
      mask help: aeroblks:aeroblkasang:blockDynamicPressureDesc
      mask init:
      | aeroicon('aeroblk');
      mask Help: eval('asbhelp');
      mask Display:
      | port_label('input',1,'V','texmode','on');
      | port_label('input',2,'\rho','texmode','on');
      | port_label('output',1,'q','texmode','on');
      | str = aeroimage('dynpres',gcb);
      | disp(str,'texmode','on');
  Mach Number : aerolibasang/Mach Number
  To Workspace1 : ToWorkspace  VariableName=vbb  SampleTime=-1
      settings: Save2DSignal=2-D array (concatenate along first dimension)
  AirData : Outport
  wires:
  Bus Creator/1 -> AirData/1
  " "/1 -> Bus Creator/1  "alpha"
  Rho/1 -> Dynamic Pressure动压/2(Air Density)
  " "/3 -> Bus Creator/3  "airpseed"
  Dynamic Pressure动压/1(qbar) -> Bus Creator/4  "q"
  " "/2 -> Bus Creator/2  "beta"
  Mach Number/1 -> Bus Creator/5  "Ma"
  Vb/1 -> Mach Number/1, Dynamic Pressure动压/1(Velocity), To Workspace1/1, " "/1
  Speed of Sound/1 -> Mach Number/2

== system simModel2020/PlantModel/B747 Dynamics动力学参数计算/Forces and Moments动力学计算/Compute Body Frame Forces and Moments气动力和力矩 ==
  AirData : Inport
  CtrlSurfaces : Inport  Port=2
  p,q,r : Inport  Port=3
  Deviation On : Inport  Port=4
  Bus Selector : BusSelector  OutputSignals=alpha,beta
  Mux : Mux  Inputs=2
  Rotate FM to body frame : Subsystem
  Wind frame F& M 气动力计算 : Subsystem
  F_b : Outport
  M_b : Outport  Port=2
  wires:
  Mux/1 -> Rotate FM to body frame/2(alpha_beta)
  Bus Selector/2 -> Mux/2  "<beta>"
  Bus Selector/1 -> Mux/1  "<alpha>"
  Wind frame F& M 气动力计算/1(FM_w) -> Rotate FM to body frame/1(FM_w)  "FM_W"
  p,q,r/1 -> Wind frame F& M 气动力计算/3(p,q,r)
  Rotate FM to body frame/2(M_b) -> M_b/1
  Rotate FM to body frame/1(F_b) -> F_b/1
  CtrlSurfaces/1 -> Wind frame F& M 气动力计算/2(CtrlSurfaces)
  AirData/1 -> Bus Selector/1, Wind frame F& M 气动力计算/1(Airdata)
  Deviation On/1 -> Wind frame F& M 气动力计算/4(Deviation On)

== system simModel2020/PlantModel/B747 Dynamics动力学参数计算/Forces and Moments动力学计算/Engine Model ==
  note: 转速
  note: 推力
  note: 燃油速率
  dt : Inport
  Ma : Inport  Port=2
  altitude : Inport  Port=3
  " Turbofan Engine System" : Subsystem  mask{IC=0, Fmax=B747.engin.MaxThrust, tau=B747.engine.static, SFC=B747.engine.fuelcon, Nt=B747.engine.ratio}
      mask prompts: IC "Initial thrust"; Fmax "Maximum sea-level static thrust"; tau "Fastest engine time constant at sea-level static (sec)"; SFC "Sea-level static thrust specific fuel consumption"; Nt "Ratio of installed thrust to uninstalled thrust"
      mask DialogControl DescGroupVar Prompt: Turbofan Engine System
      mask DialogControl DescTextVar Prompt: Implement a turbofan engine system. The turbofan engine system includes both engine and controller.  Throttle position can vary from zero to one, corresponding to no and full throttle.  Altitude, initial thrust, and maximum thrust are entered in the same unit system as selected from the block for thrust and fuel flow output.
  Constant4 : Constant  Value=0
      settings: AttributesFormatString=%<Value>
  Gain : Gain  Gain=4
  Gain1 : Gain  Gain=4
  Mux1 : Mux  Inputs=3
  N1 : Outport
  Fq : Outport  Port=2
  Thrust_b : Outport  Port=3
  wires:
  Constant4/1 -> Mux1/2, Mux1/3
  Mux1/1 -> Thrust_b/1
  " Turbofan Engine System"/1(Thrust(N)) -> Gain/1
  Gain/1 -> Mux1/1  "Thrust"
  " Turbofan Engine System"/2(Fuel flow(kg/s)) -> Gain1/1
  dt/1 -> " Turbofan Engine System"/1(Throttle_cmd)
  Ma/1 -> " Turbofan Engine System"/2(Mach)
  altitude/1 -> " Turbofan Engine System"/3(Altitude)
  Gain1/1 -> Fq/1
  " Turbofan Engine System"/3(N1) -> N1/1

== system simModel2020/PlantModel/B747 Dynamics动力学参数计算/Forces and Moments动力学计算/Rotate Vw ==
  Vw : Inport
  Euler : Inport  Port=2
  RL2B : Subsystem
  RL2B * Vw : Product  Multiplication=Matrix(*)  InputSameDT=on  SaturateOnIntegerOverflow=on  OutDataTypeStr=Inherit: Same as first input
  Vb : Outport
  wires:
  RL2B * Vw/1 -> Vb/1
  Vw/1 -> RL2B * Vw/2
  RL2B/1(RL2B) -> RL2B * Vw/1
  Euler/1 -> RL2B/1(Euler)

== system simModel2020/PlantModel/B747 Dynamics动力学参数计算/Forces and Moments动力学计算/Rotate g to Body Frame ==
  Euler : Inport
  Gravity Force : Inport  Port=2  PortDimensions=3
  Product1 : Product  Multiplication=Matrix(*)  InputSameDT=on  SaturateOnIntegerOverflow=on  OutDataTypeStr=Inherit: Same as first input
  RL2B : Subsystem
  g_b : Outport
  wires:
  Gravity Force/1 -> Product1/2
  Euler/1 -> RL2B/1(Euler)
  Product1/1 -> g_b/1
  RL2B/1(RL2B) -> Product1/1

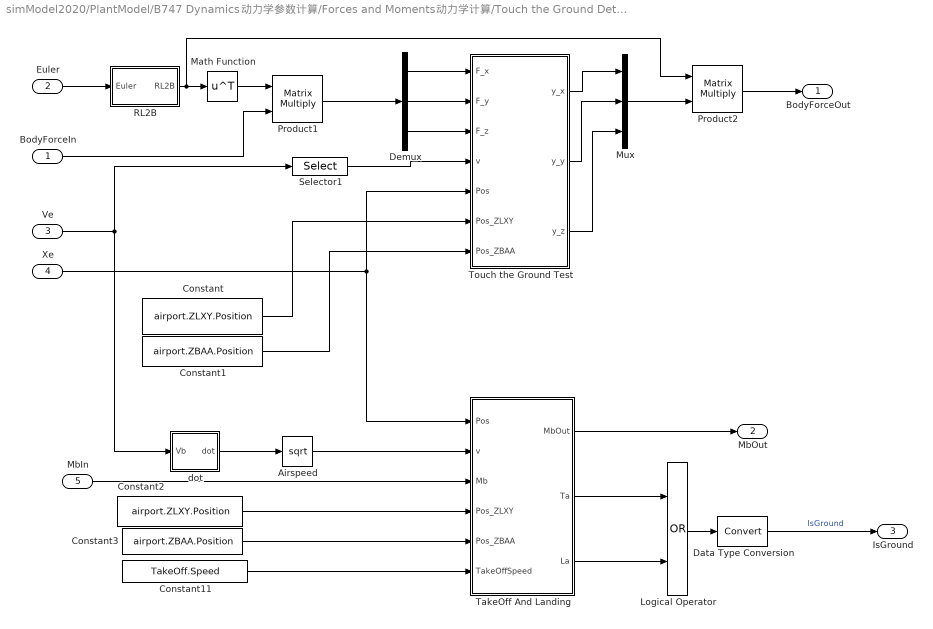
== system simModel2020/PlantModel/B747 Dynamics动力学参数计算/Forces and Moments动力学计算/Touch the Ground Detection ==
  BodyForceIn : Inport  PortDimensions=3
  Euler : Inport  Port=2
  Ve : Inport  Port=3  PortDimensions=3
  Xe : Inport  Port=4  PortDimensions=3
  MbIn : Inport  Port=5  PortDimensions=3
  Airspeed : Sqrt  AlgorithmType=Newton-Raphson
  Constant : Constant  Value=airport.ZLXY.Position
  Constant1 : Constant  Value=airport.ZBAA.Position
  Constant11 : Constant  Value=TakeOff.Speed
  Constant2 : Constant  Value=airport.ZLXY.Position
  Constant3 : Constant  Value=airport.ZBAA.Position
  Data Type Conversion : DataTypeConversion  SaturateOnIntegerOverflow=off  RndMeth=Floor
  Demux : Demux  Outputs=3
  Logical Operator : Logic  Operator=OR  AllPortsSameDT=off  OutDataTypeStr=boolean
  Math Function : Math  Operator=transpose  SignedPower=on
  Mux : Mux  Inputs=3
  Product1 : Product  Multiplication=Matrix(*)  InputSameDT=on  SaturateOnIntegerOverflow=on  OutDataTypeStr=Inherit: Same as first input
  Product2 : Product  Multiplication=Matrix(*)  InputSameDT=on  SaturateOnIntegerOverflow=on  OutDataTypeStr=Inherit: Same as first input
  RL2B : Subsystem
  Selector1 : Selector  InputPortWidth=3  IndexOptions=Index vector (dialog)  Indices=[3]  OutputSizes=1
  TakeOff And Landing : MATLAB Function  TreatAsAtomicUnit=on
  Touch the Ground Test : MATLAB Function  TreatAsAtomicUnit=on
  dot : Subsystem
  BodyForceOut : Outport
  MbOut : Outport  Port=2
  IsGround : Outport  Port=3
  wires:
  RL2B/1(RL2B) -> Product2/1, Math Function/1
  Euler/1 -> RL2B/1(Euler)
  BodyForceIn/1 -> Product1/2
  Math Function/1 -> Product1/1
  Selector1/1 -> Touch the Ground Test/4(v)
  Ve/1 -> dot/1(Vb), Selector1/1
  Product2/1 -> BodyForceOut/1
  Touch the Ground Test/3(y_z) -> Mux/3
  Product1/1 -> Demux/1
  Demux/3 -> Touch the Ground Test/3(F_z)
  Mux/1 -> Product2/2
  Constant3/1 -> TakeOff And Landing/5(Pos_ZBAA)
  Constant2/1 -> TakeOff And Landing/4(Pos_ZLXY)
  dot/1(dot) -> Airspeed/1
  MbIn/1 -> TakeOff And Landing/3(Mb)
  Constant11/1 -> TakeOff And Landing/6(TakeOffSpeed)
  Demux/1 -> Touch the Ground Test/1(F_x)
  Touch the Ground Test/1(y_x) -> Mux/1
  Demux/2 -> Touch the Ground Test/2(F_y)
  Touch the Ground Test/2(y_y) -> Mux/2
  TakeOff And Landing/1(MbOut) -> MbOut/1
  Xe/1 -> TakeOff And Landing/1(Pos), Touch the Ground Test/5(Pos)
  Airspeed/1 -> TakeOff And Landing/2(v)
  Logical Operator/1 -> Data Type Conversion/1
  Data Type Conversion/1 -> IsGround/1  "IsGround"
  TakeOff And Landing/2(Ta) -> Logical Operator/1
  TakeOff And Landing/3(La) -> Logical Operator/2
  Constant/1 -> Touch the Ground Test/6(Pos_ZLXY)
  Constant1/1 -> Touch the Ground Test/7(Pos_ZBAA)

== system simModel2020/PlantModel/Sensor Model/Assemble GPS and State Data/LLA Position ==
  XYZ (NEU) : Inport
  Display : Display
  Display1 : Display
  Flat Earth to LLA1 : aerolibtransform2/Flat Earth to LLA  units=Metric (MKS)  ptype=Earth (WGS84)  F=1/298.257223563  R=6378137  refPosPort=off  LL0=B747.ic.gsLL  psi=0
  Mux : Mux  Inputs=2
  Zero level trust : Constant  Value=0
      settings: AttributesFormatString=%<Value>
  LLA : Outport
  wires:
  Flat Earth to LLA1/1 -> Mux/1  "gps_latLon"
  Zero level trust/1 -> Flat Earth to LLA1/2
  XYZ (NEU)/1 -> Display1/1, Flat Earth to LLA1/1
  Flat Earth to LLA1/2 -> Mux/2  "gps_h"
  Mux/1 -> Display/1, LLA/1

== system simModel2020/PlantModel/Wind Model/Vonkarman Turbulence/Filters on velocities ==
  Noise : Inport
  L_ug : Inport  Port=2
  L_vg : Inport  Port=3
  L_wg : Inport  Port=4
  sigma_ug : Inport  Port=5
  sigma_vg : Inport  Port=6
  sigma_wg : Inport  Port=7
  V : Inport  Port=8
  Constant : Constant  Value=T_on
  Demux : Demux  Outputs=3
  Gu(s) : Subsystem
  Gv(s) : Subsystem
  Gw(s) : Subsystem
  ugw : Outport  OutputWhenDisabled=reset  InitialOutput=0
  vgw : Outport  Port=2  OutputWhenDisabled=reset  InitialOutput=0
  wgw : Outport  Port=3  OutputWhenDisabled=reset  InitialOutput=0
  wires:
  Demux/3 -> Gw(s)/4(Noise2)
  Constant/1 -> Gw(s)/Enable, Gv(s)/Enable, Gu(s)/Enable
  L_ug/1 -> Gu(s)/2(L_ug)
  Gu(s)/1(ugw) -> ugw/1
  Noise/1 -> Demux/1
  V/1 -> Gv(s)/3(V1), Gw(s)/1(V2), Gu(s)/1(V)
  Demux/1 -> Gu(s)/4(Noise)
  sigma_vg/1 -> Gv(s)/1(sigma_vg)
  sigma_ug/1 -> Gu(s)/3(sigma_ug)
  Demux/2 -> Gv(s)/4(Noise1)
  L_vg/1 -> Gv(s)/2(L_vg)
  L_wg/1 -> Gw(s)/2(L_wg)
  sigma_wg/1 -> Gw(s)/3(sigma_wg)
  Gv(s)/1(vgw) -> vgw/1
  Gw(s)/1(wgw) -> wgw/1

== system simModel2020/PlantModel/Wind Model/Vonkarman Turbulence/Turbulence scale lengths ==
  Altitude : Inport
  Low altitude scale length : Subsystem
  Lv : Gain  SaturateOnIntegerOverflow=on  OutDataTypeStr=Inherit: Same as input  ParamDataTypeStr=Inherit: Same as input
  Lw : Gain  SaturateOnIntegerOverflow=on  OutDataTypeStr=Inherit: Same as input  ParamDataTypeStr=Inherit: Same as input
  Mux1 : Mux  Inputs=2
  Mux2 : Mux  Inputs=2
  Subsystem : Subsystem
  L_ug : Outport
  L_vg : Outport  Port=2
  L_wg : Outport  Port=3
  wires:
  Altitude/1 -> Low altitude scale length/1(h)
  Mux2/1 -> L_ug/1, Lv/1  "Lug"
  Lv/1 -> L_vg/1
  Lw/1 -> L_wg/1
  Low altitude scale length/1(L_ug L_vg) -> Mux2/1
  Low altitude scale length/2(L_wg) -> Mux1/1
  Subsystem/1(L_ug L_vg L_wg) -> Mux1/2, Mux2/2
  Mux1/1 -> Lw/1  "Lwg"

== system simModel2020/AutoPilot/InnerLoopAutopilot/Latitudinal Channel维度通道/Lateral Correction/Filter1 ==
  x : Inport
  SW_x(k-1) : Inport  Port=2
  time : Inport  Port=3
  Constant : Constant  SampleTime=-1
  Data Type Conversion : DataTypeConversion  SaturateOnIntegerOverflow=off  RndMeth=Floor
  Detect Change : simulink/Logic and Bit Operations/Detect Change  vinit=0  OutDataTypeStr=boolean
  Gain : Gain  Gain=0.5
  Math Function : Math  SignedPower=on
  Product : Product
  Product1 : Product
  Subsystem : Subsystem
      mask Display: disp('S/H')
  Sum : Sum  Inputs=|+-
  Sum1 : Sum  Inputs=|++
  Sum2 : Sum  Inputs=+-|
  y : Outport
  wires:
  Detect Change/1 -> Subsystem/Enable
  Constant/1 -> Detect Change/1, Sum/1
  Data Type Conversion/1 -> y/1
  Sum/1 -> Product1/2
  Math Function/1 -> Sum/2, Product/1
  Gain/1 -> Math Function/1
  Sum2/1 -> Gain/1
  Subsystem/1(" ") -> Sum2/1
  time/1 -> Sum2/2, Subsystem/1(In)
  Sum1/1 -> Data Type Conversion/1
  x/1 -> Product1/1
  Product1/1 -> Sum1/1
  SW_x(k-1)/1 -> Product/2
  Product/1 -> Sum1/2

== system simModel2020/AutoPilot/InnerLoopAutopilot/Latitudinal Channel维度通道/Roll Control/Filter1 ==
  x : Inport
  SW_x(k-1) : Inport  Port=2
  time : Inport  Port=3
  Constant : Constant  SampleTime=-1
  Data Type Conversion : DataTypeConversion  SaturateOnIntegerOverflow=off  RndMeth=Floor
  Detect Change : simulink/Logic and Bit Operations/Detect Change  vinit=0  OutDataTypeStr=boolean
  Gain : Gain  Gain=0.5
  Math Function : Math  SignedPower=on
  Product : Product
  Product1 : Product
  Subsystem : Subsystem
      mask Display: disp('S/H')
  Sum : Sum  Inputs=|+-
  Sum1 : Sum  Inputs=|++
  Sum2 : Sum  Inputs=+-|
  y : Outport
  wires:
  Product/1 -> Sum1/2
  SW_x(k-1)/1 -> Product/2
  Product1/1 -> Sum1/1
  x/1 -> Product1/1
  Sum1/1 -> Data Type Conversion/1
  time/1 -> Subsystem/1(In), Sum2/2
  Subsystem/1(" ") -> Sum2/1
  Sum2/1 -> Gain/1
  Gain/1 -> Math Function/1
  Math Function/1 -> Product/1, Sum/2
  Sum/1 -> Product1/2
  Data Type Conversion/1 -> y/1
  Constant/1 -> Sum/1, Detect Change/1
  Detect Change/1 -> Subsystem/Enable

== system simModel2020/AutoPilot/InnerLoopAutopilot/Latitudinal Channel维度通道/Sample(1//z)/Detect Change ==
  note: Edge
  note: U(k)
  U : Inport
  Delay Input1 : UnitDelay  Description=Store in Global RAM  DisableCoverage=on  InitialCondition=vinit  SampleTime=-1  HasFrameUpgradeWarning=on
  FixPt Relational Operator : RelationalOperator  Operator=~=  OutDataTypeStr=boolean  ZeroCross=off  InputSameDT=off
  Y : Outport  InitialOutput=0
  wires:
  FixPt Relational Operator/1 -> Y/1
  Delay Input1/1 -> FixPt Relational Operator/2  "U(k-1)"
  U/1 -> FixPt Relational Operator/1, Delay Input1/1

== system simModel2020/AutoPilot/InnerLoopAutopilot/Latitudinal Channel维度通道/Sample(1//z)/Sample and Hold ==
  In : Inport
  Trigger : TriggerPort  TriggerType=either  VariantControl=Variant  ZeroCross=off
  " " : Outport  InitialOutput=initCond
  wires:
  In/1 -> " "/1
